simulink model "ASSIGNMEMT"  (R2020b)
settings: Solver=FixedStepAuto  StartTime=0.0  StopTime=1.5  FixedStep=0.000001  RelTol=1e-3
settings Model: NumberOfSteps=50  Creator=99714  LastModifiedBy=99714
settings OptimizationCC: DefaultParameterBehavior=Inlined  EnhancedBackFolding=on  PassReuseOutputArgsAs=Individual arguments  ZeroExternalMemoryAtStartup=off  ZeroInternalMemoryAtStartup=off  OptimizeBlockOrder=speed  DifferentSizesBufferReuse=on  OptimizationCustomize=off  EfficientTunableParamExpr=on
settings DebuggingCC: ParameterTunabilityLossMsg=error
settings SFSimCC: MATLABDynamicMemAlloc=off
settings RTWCC: Description=Embedded Coder  SystemTargetFile=ert.tlc  GenCodeOnly=on  TemplateMakefile=ert_default_tmf  GenerateReport=on  LaunchReport=on
settings CodeAppCC: ForceParamTrailComments=on  IgnoreCustomStorageClasses=off  OperatorAnnotations=on  SimulinkDataObjDesc=on  SFDataObjDesc=on  InsertBlockDesc=on
settings ERTTargetCC: TargetLangStandard=C99 (ISO)  GenerateSampleERTMain=on  InlinedParameterPlacement=NonHierarchical  ERTCustomFileTemplate=example_file_process.tlc  ERTFilePackagingFormat=Compact

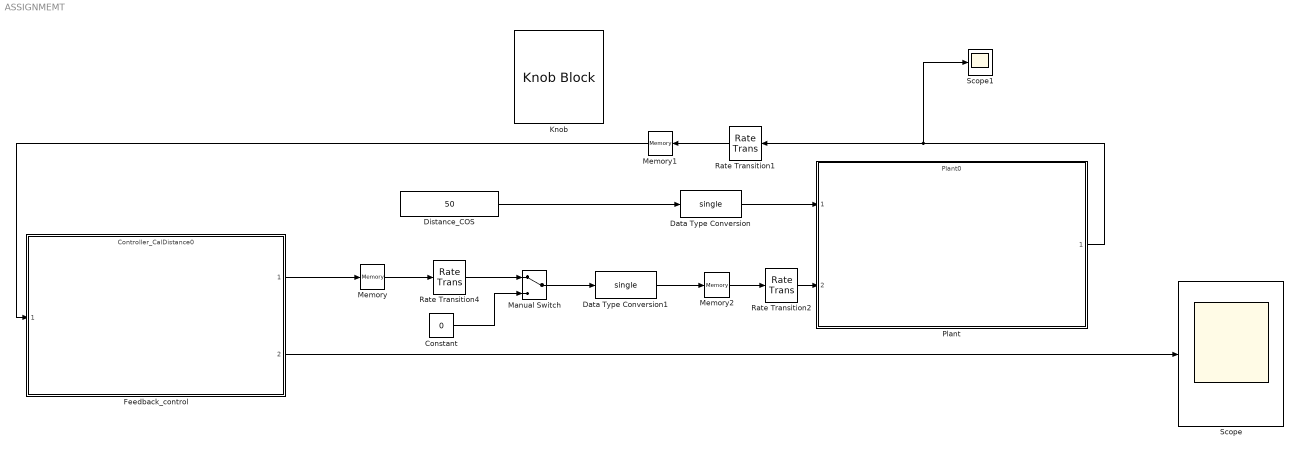
== system ASSIGNMEMT ==
  Constant : Constant  Value=0
  Data Type Conversion : DataTypeConversion  OutDataTypeStr=single
  Data Type Conversion1 : DataTypeConversion  OutDataTypeStr=single
  Distance_COS : Constant  Value=50
  Feedback_control : ModelReference  ModelNameDialog=Controller_CalDistance0  SimulationMode=Normal  ModelReferenceVersion=1.46
  Knob : KnobBlock  ScaleMin=2  ScaleMax=400
  Manual Switch : ManualSwitch
  Memory : Memory
  Memory1 : Memory
  Memory2 : Memory
  Plant : ModelReference  ModelNameDialog=Plant0  SimulationMode=Normal  ModelReferenceVersion=1.24
  Rate Transition1 : RateTransition
  Rate Transition2 : RateTransition
  Rate Transition4 : RateTransition
  Scope : Scope
  Scope1 : Scope
  wires:
  Distance_COS/1 -> Data Type Conversion/1
  Constant/1 -> Manual Switch/2
  Manual Switch/1 -> Data Type Conversion1/1
  Feedback_control/2 -> Scope/1
  Data Type Conversion/1 -> Plant/1
  Plant/1 -> Scope1/1, Rate Transition1/1
  Rate Transition4/1 -> Manual Switch/1
  Rate Transition1/1 -> Memory1/1
  Rate Transition2/1 -> Plant/2
  Feedback_control/1 -> Memory/1
  Memory/1 -> Rate Transition4/1
  Memory1/1 -> Feedback_control/1
  Data Type Conversion1/1 -> Memory2/1
  Memory2/1 -> Rate Transition2/1
